simulink model "SIL_Simulation_Position_Control"  (R2022b)
settings: Solver=FixedStepAuto  StartTime=0.0  StopTime=18  RelTol=1e-3
undefined symbols (not defined in the file): Ad, Bd, Cd, Dd, Ts
settings Model: Creator=Marco  LastModifiedBy=Marco
settings OptimizationCC: ReuseModelBlockBuffer=on

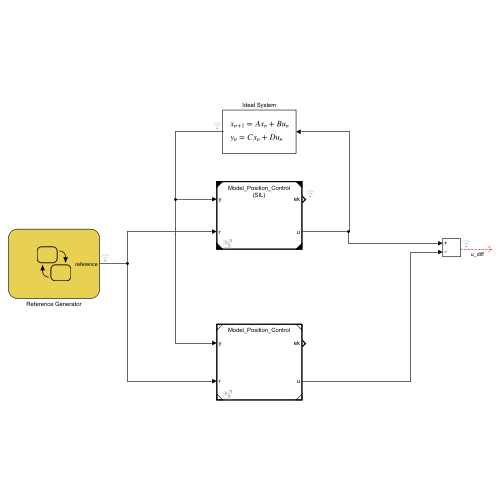
[thumbnail: Simulink's stored preview of the top-level diagram]
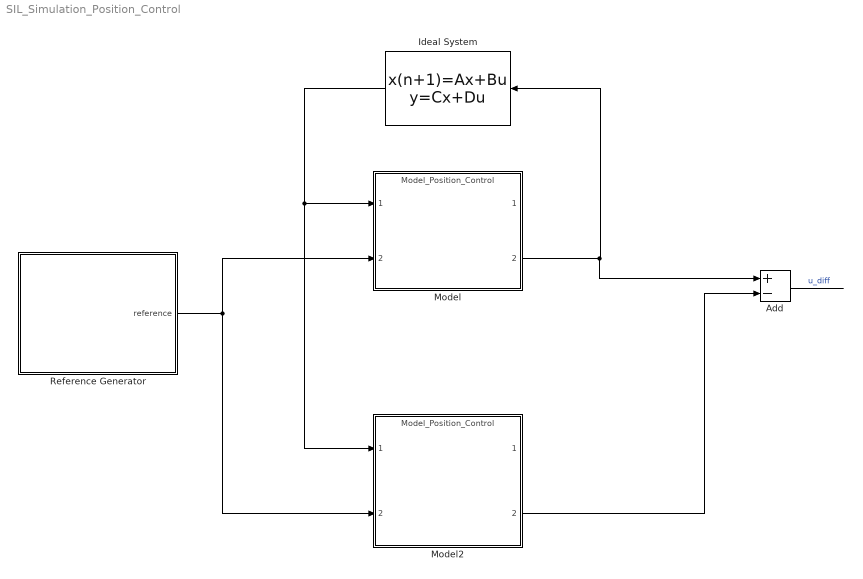
== system SIL_Simulation_Position_Control ==
  Add : Sum  Inputs=+-
  Ideal System : DiscreteStateSpace  A=Ad  B=Bd  C=Cd  D=Dd  SampleTime=Ts
  Model : ModelReference  ModelNameDialog=Model_Position_Control.slx  SimulationMode=Software-in-the-loop (SIL)  ModelReferenceVersion=1.12
  Model2 : ModelReference  ModelNameDialog=Model_Position_Control.slx  SimulationMode=Normal  ModelReferenceVersion=1.12
  Reference Generator : Stateflow chart  TreatAsAtomicUnit=on
  wires:
  Ideal System/1 -> Model2/1, Model/1
  Reference Generator/1(reference) -> Model2/2, Model/2
  Add/1 -> ?  "u_diff"
  Model2/2 -> Add/2
  Model/2 -> Ideal System/1, Add/1

== stateflow chart SIL_Simulation_Position_Control/Reference Generator ==
  state Start
    reference = 0;
  state State1
    reference = deg2rad(30)
  state State4
    reference = deg2rad(-30)
  state State2
    reference = deg2rad(720)
  state State3
    reference = deg2rad(-720)
  state State5
    reference = 0
  (default) -> Start
  Start -> State1 : [after(4,sec)]
  State1 -> State4 : [after(4,sec)]
  State4 -> State2 : [after(4,sec)]
  State3 -> Start : [after(4,sec)]
  State2 -> State5 : [after(4,sec)]
  State5 -> State3 : [after(4,sec)]
  data: reference output
